simulink model "simulink_testbench"  (R2025b)
settings: Solver=VariableStepAuto  StartTime=0.0  StopTime=1.1  RelTol=1e-3
settings Model: Creator=Sarthak  LastModifiedBy=Sarthak

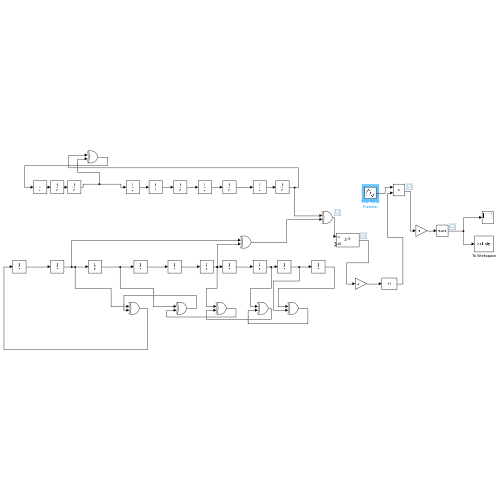
[thumbnail: Simulink's stored preview of the top-level diagram]
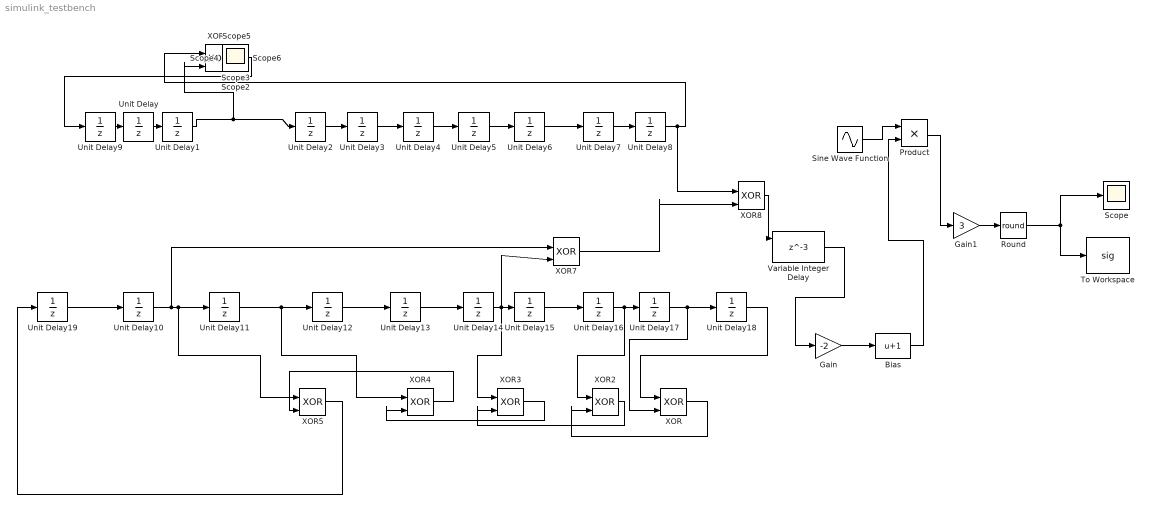
== system simulink_testbench ==
  Bias : Bias  Bias=1  SaturateOnIntegerOverflow=off
  Gain : Gain  Gain=-2
  Gain1 : Gain  Gain=3
  Product : Product
  Round : Rounding  Operator=round
  Scope{,1..6} (7 alike) : Scope
      Scope1 settings: ActiveDisplayYMinimum=-0.57191115145358629  ActiveDisplayYMaximum=2.6378917940205291
      Scope2 settings: ActiveDisplayYMinimum=-0.15356347079891114  ActiveDisplayYMaximum=1.1751984001677263  DataLoggingVariableName=ScopeData2
      Scope3 settings: ActiveDisplayYMinimum=-0.12499999999999997  ActiveDisplayYMaximum=1.125  DataLoggingVariableName=ScopeData3
      Scope4 settings: ActiveDisplayYMinimum=-0.12499999999999997  ActiveDisplayYMaximum=1.125  DataLoggingVariableName=ScopeData4
      Scope5 settings: ActiveDisplayYMinimum=-1.2499997391869795  ActiveDisplayYMaximum=1.2499997538603465  DataLoggingVariableName=ScopeData5
      Scope6 settings: ActiveDisplayYMinimum=-3.75  ActiveDisplayYMaximum=3.75  DataLoggingVariableName=ScopeData6
  Sine Wave Function : Sin  Frequency=9250000  SampleTime=0
  To Workspace : ToWorkspace  VariableName=sig  SampleTime=-1
      settings: Save2DSignal=2-D array (concatenate along first dimension)
  Unit Delay{,1..19} (20 alike) : UnitDelay  InitialCondition=1  SampleTime=9.775E-7  HasFrameUpgradeWarning=on
  Variable Integer Delay : Delay  DelayLength=3  InitialConditionSource=Input port  SampleTime=1
      settings: InputPortMap=u0,p4
  XOR{,1..5,7..8} (8 alike) : Logic  Operator=XOR  IconShape=distinctive  AllPortsSameDT=off  OutDataTypeStr=boolean
  wires:
  Unit Delay1/1 -> XOR1/2, Unit Delay2/1
  Unit Delay/1 -> Unit Delay1/1
  Unit Delay3/1 -> Unit Delay4/1
  Unit Delay2/1 -> Unit Delay3/1
  Unit Delay9/1 -> Unit Delay/1
  Unit Delay4/1 -> Unit Delay5/1
  Unit Delay5/1 -> Unit Delay6/1
  Unit Delay6/1 -> Unit Delay7/1
  Unit Delay7/1 -> Unit Delay8/1
  Unit Delay13/1 -> Unit Delay14/1
  Unit Delay15/1 -> Unit Delay16/1
  Unit Delay12/1 -> Unit Delay13/1
  Unit Delay16/1 -> XOR2/1, Unit Delay17/1
  Unit Delay19/1 -> Unit Delay10/1
  Unit Delay14/1 -> XOR3/1, XOR7/2, Unit Delay15/1
  Unit Delay17/1 -> XOR/2, Unit Delay18/1
  Unit Delay11/1 -> XOR4/1, Unit Delay12/1
  Unit Delay10/1 -> XOR7/1, XOR5/1, Unit Delay11/1
  Unit Delay8/1 -> XOR8/1, XOR1/1
  XOR1/1 -> Unit Delay9/1
  Unit Delay18/1 -> XOR/1
  XOR/1 -> XOR2/2
  XOR2/1 -> XOR3/2
  XOR3/1 -> XOR4/2
  XOR4/1 -> XOR5/2
  XOR5/1 -> Unit Delay19/1
  XOR7/1 -> XOR8/2
  XOR8/1 -> Variable Integer Delay/1
  Sine Wave Function/1 -> Product/1
  Variable Integer Delay/1 -> Gain/1
  Product/1 -> Gain1/1
  Gain/1 -> Bias/1
  Bias/1 -> Product/2
  Gain1/1 -> Round/1
  Round/1 -> To Workspace/1, Scope/1
